simulink model "Vorlage_Anlagenteil_Pruefen_Jaehocha"  (R2021b)
settings: Solver=ode3  StartTime=0.0  StopTime=50  FixedStep=0.01  RelTol=1e-3
StopFcn:
  | clear con
model workspace (MAT data in the model file):
  A : Simulink.Signal (value not decoded)
undefined symbols (not defined in the file): sigbuilder_block
libraries: simulink x10, simulink_extras x7, aerolibanimutils x1
(part 2 of 2)

== system Vorlage_Anlagenteil_Pruefen_Jaehocha/Systemtest Simulation1/2_rot_mit_Deckel/Signal Builder10 ==
  Demux : Demux  Tag=STV Demux  Outputs=8
      settings: DisplayOption=none
  FromWs : FromWorkspace  Tag=STV FromWs  VariableName=tuvar
      SigBuilderData=|
      | common.afterFinalStr = 'Extrapolate'
      | common.sampleTime = 0
      | dataSet.timeRange = [0 11]
      | dataSet.name = 'Group 1'
      | sbobj.Groups.Name = 'Group 1'
      | sbobj.Groups.Signals(1).Name = 'aufzug_abwaerts'
      | sbobj.Groups.Signals(1).XData = [0 6 6 10.5 10.5 11]
      | sbobj.Groups.Signals(1).YData = [0 0 1 1 0 0]
      | sbobj.Groups.Signals(2).Name = 'aufzug_aufwaerts'
      | sbobj.Groups.Signals(2).XData = [0 0.5 0.5 5 5 11]
      | sbobj.Groups.Signals(2).YData = [0 0 1 1 0 0]
      | sbobj.Groups.Signals(3).Name = 'zylinder_ausschieben'
      | sbobj.Groups.Signals(3).XData = [0 5.5 5.5 6.2 6.2 11]
      | sbobj.Groups.Signals(3).YData = [0 0 1 1 0 0]
      | sbobj.Groups.Signals(4).Name = 'luft_an'
      | sbobj.Groups.Signals(4).XData = [0 5.5 5.5 7.5 7.5 11]
      | sbobj.Groups.Signals(4).YData = [0 0 1 1 0 0]
      | sbobj.Groups.Signals(5).Name = 'Signal 5'
      | sbobj.Groups.Signals(5).XData = [0 11]
      | sbobj.Groups.Signals(5).YData = [0 0]
      | sbobj.Groups.Signals(6).Name = 'Signal 6'
      | sbobj.Groups.Signals(6).XData = [0 11]
      | sbobj.Groups.Signals(6).YData = [0 0]
      | sbobj.Groups.Signals(7).Name = 'Signal 7'
      | sbobj.Groups.Signals(7).XData = [0 11]
      | sbobj.Groups.Signals(7).YData = [0 0]
      | sbobj.Groups.Signals(8).Name = 'station_frei'
      | sbobj.Groups.Signals(8).XData = [0 0.1 0.1 11]
      | sbobj.Groups.Signals(8).YData = [1 1 0 0]
      | sbobj.Groups.TimeRange = [0 11]
  aufzug_abwaerts : Outport  Tag=STV Outport  VectorParamsAs1DForOutWhenUnconnected=off
  aufzug_aufwaerts : Outport  Tag=STV Outport  Port=2  VectorParamsAs1DForOutWhenUnconnected=off
  zylinder_ausschieben : Outport  Tag=STV Outport  Port=3  VectorParamsAs1DForOutWhenUnconnected=off
  luft_an : Outport  Tag=STV Outport  Port=4  VectorParamsAs1DForOutWhenUnconnected=off
  Signal 5 : Outport  Tag=STV Outport  Port=5  VectorParamsAs1DForOutWhenUnconnected=off
  Signal 6 : Outport  Tag=STV Outport  Port=6  VectorParamsAs1DForOutWhenUnconnected=off
  Signal 7 : Outport  Tag=STV Outport  Port=7  VectorParamsAs1DForOutWhenUnconnected=off
  station_frei : Outport  Tag=STV Outport  Port=8  VectorParamsAs1DForOutWhenUnconnected=off
  wires:
  Demux/1 -> aufzug_abwaerts/1
  FromWs/1 -> Demux/1
  Demux/2 -> aufzug_aufwaerts/1
  Demux/3 -> zylinder_ausschieben/1
  Demux/4 -> luft_an/1
  Demux/5 -> Signal 5/1
  Demux/6 -> Signal 6/1
  Demux/7 -> Signal 7/1
  Demux/8 -> station_frei/1

== system Vorlage_Anlagenteil_Pruefen_Jaehocha/Systemtest Simulation1/2_rot_mit_Deckel/Signal Builder4 ==
  Demux : Demux  Tag=STV Demux  Outputs=6
      settings: DisplayOption=none
  FromWs : FromWorkspace  Tag=STV FromWs  VariableName=tuvar
      SigBuilderData=|
      | common.afterFinalStr = 'Extrapolate'
      | common.sampleTime = 0
      | dataSet.timeRange = [0 11]
      | dataSet.name = 'Group 1'
      | sbobj.Groups.Name = 'Group 1'
      | sbobj.Groups.Signals(1).Name = 'zylinder_platziert'
      | sbobj.Groups.Signals(1).XData = [0 0.3 0.3 11]
      | sbobj.Groups.Signals(1).YData = [1 1 0 0]
      | sbobj.Groups.Signals(2).Name = 'zylinder_schwarz'
      | sbobj.Groups.Signals(2).XData = [0 11]
      | sbobj.Groups.Signals(2).YData = [0 0]
      | sbobj.Groups.Signals(3).Name = 'zylinder_hoehe'
      | sbobj.Groups.Signals(3).XData = [0 5 5 5.6 5.6 11]
      | sbobj.Groups.Signals(3).YData = [0 0 28 28 0 0]
      | sbobj.Groups.Signals(4).Name = 'arbeitsraum_frei'
      | sbobj.Groups.Signals(4).XData = [0 0.5 0.5 10.5 10.5 10.8 10.8 11]
      | sbobj.Groups.Signals(4).YData = [1 1 0 0 1 1 0 0]
      | sbobj.Groups.Signals(5).Name = 'zylinder_entfernt_folge'
      | sbobj.Groups.Signals(5).XData = [0 10 10 10.5 10.5 11]
      | sbobj.Groups.Signals(5).YData = [0 0 1 1 0 0]
      | sbobj.Groups.Signals(6).Name = 'folge_belegt'
      | sbobj.Groups.Signals(6).XData = [0 4 5.5 11]
      | sbobj.Groups.Signals(6).YData = [0 0 0 0]
      | sbobj.Groups.TimeRange = [0 11]
  zylinder_platziert : Outport  Tag=STV Outport  VectorParamsAs1DForOutWhenUnconnected=off
  zylinder_schwarz : Outport  Tag=STV Outport  Port=2  VectorParamsAs1DForOutWhenUnconnected=off
  zylinder_hoehe : Outport  Tag=STV Outport  Port=3  VectorParamsAs1DForOutWhenUnconnected=off
  arbeitsraum_frei : Outport  Tag=STV Outport  Port=4  VectorParamsAs1DForOutWhenUnconnected=off
  zylinder_entfernt_folge : Outport  Tag=STV Outport  Port=5  VectorParamsAs1DForOutWhenUnconnected=off
  folge_belegt : Outport  Tag=STV Outport  Port=6  VectorParamsAs1DForOutWhenUnconnected=off
  wires:
  Demux/1 -> zylinder_platziert/1
  FromWs/1 -> Demux/1
  Demux/2 -> zylinder_schwarz/1
  Demux/3 -> zylinder_hoehe/1
  Demux/4 -> arbeitsraum_frei/1
  Demux/5 -> zylinder_entfernt_folge/1
  Demux/6 -> folge_belegt/1

== system Vorlage_Anlagenteil_Pruefen_Jaehocha/Systemtest Simulation1/2_rot_mit_Deckel/arbeitsraum_frei ==
  Add : Sum  Inputs=++++
  Constant : Constant
  Constant1 : Constant  Value=-1
  Constant2 : Constant
  Constant3 : Constant  Value=-1
  Data Type Conversion : DataTypeConversion  OutDataTypeStr=boolean
  Delay : Delay  DelayLength=0
  Delay1 : Delay  DelayLength=200
  Delay2 : Delay  DelayLength=1050
  Delay3 : Delay  DelayLength=1080
  Out1 : Outport  VectorParamsAs1DForOutWhenUnconnected=off
  wires:
  Constant/1 -> Delay/1
  Constant1/1 -> Delay1/1
  Delay/1 -> Add/1
  Delay1/1 -> Add/2
  Add/1 -> Data Type Conversion/1
  Data Type Conversion/1 -> Out1/1
  Constant2/1 -> Delay2/1
  Delay2/1 -> Add/3
  Constant3/1 -> Delay3/1
  Delay3/1 -> Add/4

== system Vorlage_Anlagenteil_Pruefen_Jaehocha/Systemtest Simulation1/2_rot_mit_Deckel/aufzug_abwaerts ==
  Add : Sum
  Constant : Constant
  Constant1 : Constant  Value=-1
  Data Type Conversion : DataTypeConversion  OutDataTypeStr=boolean
  Delay : Delay  DelayLength=600
  Delay1 : Delay  DelayLength=1050
  Out1 : Outport  VectorParamsAs1DForOutWhenUnconnected=off
  wires:
  Constant/1 -> Delay/1
  Constant1/1 -> Delay1/1
  Delay/1 -> Add/1
  Delay1/1 -> Add/2
  Add/1 -> Data Type Conversion/1
  Data Type Conversion/1 -> Out1/1

== system Vorlage_Anlagenteil_Pruefen_Jaehocha/Systemtest Simulation1/2_rot_mit_Deckel/aufzug_aufwaerts ==
  Add : Sum
  Constant : Constant
  Constant1 : Constant  Value=-1
  Data Type Conversion : DataTypeConversion  OutDataTypeStr=boolean
  Delay : Delay  DelayLength=50
  Delay1 : Delay  DelayLength=500
  Out1 : Outport  VectorParamsAs1DForOutWhenUnconnected=off
  wires:
  Constant/1 -> Delay/1
  Constant1/1 -> Delay1/1
  Delay/1 -> Add/1
  Delay1/1 -> Add/2
  Add/1 -> Data Type Conversion/1
  Data Type Conversion/1 -> Out1/1

== system Vorlage_Anlagenteil_Pruefen_Jaehocha/Systemtest Simulation1/2_rot_mit_Deckel/done_signal ==
  Constant : Constant
  Data Type Conversion : DataTypeConversion  OutDataTypeStr=boolean
  Delay : Delay  DelayLength=1080
  Out1 : Outport  VectorParamsAs1DForOutWhenUnconnected=off
  wires:
  Constant/1 -> Delay/1
  Data Type Conversion/1 -> Out1/1
  Delay/1 -> Data Type Conversion/1

== system Vorlage_Anlagenteil_Pruefen_Jaehocha/Systemtest Simulation1/2_rot_mit_Deckel/folge_belegt ==
  Constant : Constant  Value=0
  Data Type Conversion : DataTypeConversion  OutDataTypeStr=boolean
  Out1 : Outport  VectorParamsAs1DForOutWhenUnconnected=off
  wires:
  Constant/1 -> Data Type Conversion/1
  Data Type Conversion/1 -> Out1/1

== system Vorlage_Anlagenteil_Pruefen_Jaehocha/Systemtest Simulation1/2_rot_mit_Deckel/luft_an ==
  Add : Sum
  Constant : Constant
  Constant1 : Constant  Value=-1
  Data Type Conversion : DataTypeConversion  OutDataTypeStr=boolean
  Delay : Delay  DelayLength=550
  Delay1 : Delay  DelayLength=750
  Out1 : Outport  VectorParamsAs1DForOutWhenUnconnected=off
  wires:
  Constant/1 -> Delay/1
  Constant1/1 -> Delay1/1
  Delay/1 -> Add/1
  Delay1/1 -> Add/2
  Add/1 -> Data Type Conversion/1
  Data Type Conversion/1 -> Out1/1

== system Vorlage_Anlagenteil_Pruefen_Jaehocha/Systemtest Simulation1/2_rot_mit_Deckel/out5 ==
  Add : Sum
  Constant : Constant
  Constant1 : Constant  Value=-1
  Data Type Conversion : DataTypeConversion  OutDataTypeStr=boolean
  Delay : Delay  DelayLength=0
  Delay1 : Delay  DelayLength=0
  Out1 : Outport  VectorParamsAs1DForOutWhenUnconnected=off
  wires:
  Constant/1 -> Delay/1
  Constant1/1 -> Delay1/1
  Delay/1 -> Add/1
  Delay1/1 -> Add/2
  Add/1 -> Data Type Conversion/1
  Data Type Conversion/1 -> Out1/1

== system Vorlage_Anlagenteil_Pruefen_Jaehocha/Systemtest Simulation1/2_rot_mit_Deckel/out6 ==
  Add : Sum
  Constant : Constant
  Constant1 : Constant  Value=-1
  Data Type Conversion : DataTypeConversion  OutDataTypeStr=boolean
  Delay : Delay  DelayLength=0
  Delay1 : Delay  DelayLength=0
  Out1 : Outport  VectorParamsAs1DForOutWhenUnconnected=off
  wires:
  Constant/1 -> Delay/1
  Constant1/1 -> Delay1/1
  Delay/1 -> Add/1
  Delay1/1 -> Add/2
  Add/1 -> Data Type Conversion/1
  Data Type Conversion/1 -> Out1/1

== system Vorlage_Anlagenteil_Pruefen_Jaehocha/Systemtest Simulation1/2_rot_mit_Deckel/out7 ==
  Add : Sum
  Constant : Constant
  Constant1 : Constant  Value=-1
  Data Type Conversion : DataTypeConversion  OutDataTypeStr=boolean
  Delay : Delay  DelayLength=0
  Delay1 : Delay  DelayLength=0
  Out1 : Outport  VectorParamsAs1DForOutWhenUnconnected=off
  wires:
  Constant/1 -> Delay/1
  Constant1/1 -> Delay1/1
  Delay/1 -> Add/1
  Delay1/1 -> Add/2
  Add/1 -> Data Type Conversion/1
  Data Type Conversion/1 -> Out1/1

== system Vorlage_Anlagenteil_Pruefen_Jaehocha/Systemtest Simulation1/2_rot_mit_Deckel/station_frei ==
  Add : Sum
  Constant : Constant
  Constant1 : Constant  Value=-1
  Data Type Conversion : DataTypeConversion  OutDataTypeStr=boolean
  Delay : Delay  DelayLength=0
  Delay1 : Delay  DelayLength=10
  Out1 : Outport  VectorParamsAs1DForOutWhenUnconnected=off
  wires:
  Constant/1 -> Delay/1
  Constant1/1 -> Delay1/1
  Delay/1 -> Add/1
  Delay1/1 -> Add/2
  Add/1 -> Data Type Conversion/1
  Data Type Conversion/1 -> Out1/1

== system Vorlage_Anlagenteil_Pruefen_Jaehocha/Systemtest Simulation1/2_rot_mit_Deckel/zylinder_ausschieben ==
  Add : Sum
  Constant : Constant
  Constant1 : Constant  Value=-1
  Data Type Conversion : DataTypeConversion  OutDataTypeStr=boolean
  Delay : Delay  DelayLength=550
  Delay1 : Delay  DelayLength=620
  Out1 : Outport  VectorParamsAs1DForOutWhenUnconnected=off
  wires:
  Constant/1 -> Delay/1
  Constant1/1 -> Delay1/1
  Delay/1 -> Add/1
  Delay1/1 -> Add/2
  Add/1 -> Data Type Conversion/1
  Data Type Conversion/1 -> Out1/1

== system Vorlage_Anlagenteil_Pruefen_Jaehocha/Systemtest Simulation1/2_rot_mit_Deckel/zylinder_entfernt_folge ==
  Add : Sum
  Constant : Constant
  Constant1 : Constant  Value=-1
  Data Type Conversion : DataTypeConversion  OutDataTypeStr=boolean
  Delay : Delay  DelayLength=1000
  Delay1 : Delay  DelayLength=1050
  Out1 : Outport  VectorParamsAs1DForOutWhenUnconnected=off
  wires:
  Constant/1 -> Delay/1
  Constant1/1 -> Delay1/1
  Delay/1 -> Add/1
  Delay1/1 -> Add/2
  Add/1 -> Data Type Conversion/1
  Data Type Conversion/1 -> Out1/1

== system Vorlage_Anlagenteil_Pruefen_Jaehocha/Systemtest Simulation1/2_rot_mit_Deckel/zylinder_hoehe ==
  Add : Sum
  Constant : Constant  Value=28
  Constant1 : Constant  Value=-28
  Delay : Delay  DelayLength=50
  Delay1 : Delay  DelayLength=900
  Out1 : Outport  VectorParamsAs1DForOutWhenUnconnected=off
  wires:
  Constant/1 -> Delay/1
  Constant1/1 -> Delay1/1
  Delay/1 -> Add/1
  Delay1/1 -> Add/2
  Add/1 -> Out1/1

== system Vorlage_Anlagenteil_Pruefen_Jaehocha/Systemtest Simulation1/2_rot_mit_Deckel/zylinder_platziert ==
  Add : Sum
  Constant : Constant
  Constant1 : Constant  Value=-1
  Data Type Conversion : DataTypeConversion  OutDataTypeStr=boolean
  Delay : Delay  DelayLength=0
  Delay1 : Delay  DelayLength=30
  Out1 : Outport  VectorParamsAs1DForOutWhenUnconnected=off
  wires:
  Constant/1 -> Delay/1
  Constant1/1 -> Delay1/1
  Delay/1 -> Add/1
  Delay1/1 -> Add/2
  Add/1 -> Data Type Conversion/1
  Data Type Conversion/1 -> Out1/1

== system Vorlage_Anlagenteil_Pruefen_Jaehocha/Systemtest Simulation1/2_rot_mit_Deckel/zylinder_schwarz ==
  Add : Sum
  Constant : Constant
  Constant1 : Constant  Value=-1
  Data Type Conversion : DataTypeConversion  OutDataTypeStr=boolean
  Delay : Delay  DelayLength=0
  Delay1 : Delay  DelayLength=0
  Out1 : Outport  VectorParamsAs1DForOutWhenUnconnected=off
  wires:
  Constant/1 -> Delay/1
  Constant1/1 -> Delay1/1
  Delay/1 -> Add/1
  Delay1/1 -> Add/2
  Add/1 -> Data Type Conversion/1
  Data Type Conversion/1 -> Out1/1

== system Vorlage_Anlagenteil_Pruefen_Jaehocha/Systemtest Simulation1/3_rot_ohne_Deckel/Signal Builder10 ==
  Demux : Demux  Tag=STV Demux  Outputs=8
      settings: DisplayOption=none
  FromWs : FromWorkspace  Tag=STV FromWs  VariableName=tuvar
      SigBuilderData=|
      | common.afterFinalStr = 'Extrapolate'
      | common.sampleTime = 0
      | dataSet.timeRange = [0 11]
      | dataSet.name = 'Group 1'
      | sbobj.Groups.Name = 'Group 1'
      | sbobj.Groups.Signals(1).Name = 'aufzug_abwaerts'
      | sbobj.Groups.Signals(1).XData = [0 5.5 5.5 10 10 11]
      | sbobj.Groups.Signals(1).YData = [0 0 1 1 0 0]
      | sbobj.Groups.Signals(2).Name = 'aufzug_aufwaerts'
      | sbobj.Groups.Signals(2).XData = [0 0.5 0.5 5 5 11]
      | sbobj.Groups.Signals(2).YData = [0 0 1 1 0 0]
      | sbobj.Groups.Signals(3).Name = 'zylinder_ausschieben'
      | sbobj.Groups.Signals(3).XData = [0 10 10 10.48 10.48 11]
      | sbobj.Groups.Signals(3).YData = [0 0 1 1 0 0]
      | sbobj.Groups.Signals(4).Name = 'luft_an'
      | sbobj.Groups.Signals(4).XData = [0 7.5 11]
      | sbobj.Groups.Signals(4).YData = [0 0 0]
      | sbobj.Groups.Signals(5).Name = 'Signal 5'
      | sbobj.Groups.Signals(5).XData = [0 11]
      | sbobj.Groups.Signals(5).YData = [0 0]
      | sbobj.Groups.Signals(6).Name = 'Signal 6'
      | sbobj.Groups.Signals(6).XData = [0 11]
      | sbobj.Groups.Signals(6).YData = [0 0]
      | sbobj.Groups.Signals(7).Name = 'Signal 7'
      | sbobj.Groups.Signals(7).XData = [0 11]
      | sbobj.Groups.Signals(7).YData = [0 0]
      | sbobj.Groups.Signals(8).Name = 'station_frei'
      | sbobj.Groups.Signals(8).XData = [0 0.1 0.1 11]
      | sbobj.Groups.Signals(8).YData = [1 1 0 0]
      | sbobj.Groups.TimeRange = [0 11]
  aufzug_abwaerts : Outport  Tag=STV Outport  VectorParamsAs1DForOutWhenUnconnected=off
  aufzug_aufwaerts : Outport  Tag=STV Outport  Port=2  VectorParamsAs1DForOutWhenUnconnected=off
  zylinder_ausschieben : Outport  Tag=STV Outport  Port=3  VectorParamsAs1DForOutWhenUnconnected=off
  luft_an : Outport  Tag=STV Outport  Port=4  VectorParamsAs1DForOutWhenUnconnected=off
  Signal 5 : Outport  Tag=STV Outport  Port=5  VectorParamsAs1DForOutWhenUnconnected=off
  Signal 6 : Outport  Tag=STV Outport  Port=6  VectorParamsAs1DForOutWhenUnconnected=off
  Signal 7 : Outport  Tag=STV Outport  Port=7  VectorParamsAs1DForOutWhenUnconnected=off
  station_frei : Outport  Tag=STV Outport  Port=8  VectorParamsAs1DForOutWhenUnconnected=off
  wires:
  Demux/1 -> aufzug_abwaerts/1
  FromWs/1 -> Demux/1
  Demux/2 -> aufzug_aufwaerts/1
  Demux/3 -> zylinder_ausschieben/1
  Demux/4 -> luft_an/1
  Demux/5 -> Signal 5/1
  Demux/6 -> Signal 6/1
  Demux/7 -> Signal 7/1
  Demux/8 -> station_frei/1

== system Vorlage_Anlagenteil_Pruefen_Jaehocha/Systemtest Simulation1/3_rot_ohne_Deckel/Signal Builder4 ==
  Demux : Demux  Tag=STV Demux  Outputs=6
      settings: DisplayOption=none
  FromWs : FromWorkspace  Tag=STV FromWs  VariableName=tuvar
      SigBuilderData=|
      | common.afterFinalStr = 'Extrapolate'
      | common.sampleTime = 0
      | dataSet.timeRange = [0 11]
      | dataSet.name = 'Group 1'
      | sbobj.Groups.Name = 'Group 1'
      | sbobj.Groups.Signals(1).Name = 'zylinder_platziert'
      | sbobj.Groups.Signals(1).XData = [0 0.3 0.3 11]
      | sbobj.Groups.Signals(1).YData = [1 1 0 0]
      | sbobj.Groups.Signals(2).Name = 'zylinder_schwarz'
      | sbobj.Groups.Signals(2).XData = [0 11]
      | sbobj.Groups.Signals(2).YData = [0 0]
      | sbobj.Groups.Signals(3).Name = 'zylinder_hoehe'
      | sbobj.Groups.Signals(3).XData = [0 5 5 5.6 5.6 11]
      | sbobj.Groups.Signals(3).YData = [0 0 25 25 0 0]
      | sbobj.Groups.Signals(4).Name = 'arbeitsraum_frei'
      | sbobj.Groups.Signals(4).XData = [0 0.5 0.5 10 10 10.8 10.8 11]
      | sbobj.Groups.Signals(4).YData = [1 1 0 0 1 1 0 0]
      | sbobj.Groups.Signals(5).Name = 'zylinder_entfernt_folge'
      | sbobj.Groups.Signals(5).XData = [0 10 10.5 11]
      | sbobj.Groups.Signals(5).YData = [0 0 0 0]
      | sbobj.Groups.Signals(6).Name = 'folge_belegt'
      | sbobj.Groups.Signals(6).XData = [0 4 5.5 11]
      | sbobj.Groups.Signals(6).YData = [0 0 0 0]
      | sbobj.Groups.TimeRange = [0 11]
  zylinder_platziert : Outport  Tag=STV Outport  VectorParamsAs1DForOutWhenUnconnected=off
  zylinder_schwarz : Outport  Tag=STV Outport  Port=2  VectorParamsAs1DForOutWhenUnconnected=off
  zylinder_hoehe : Outport  Tag=STV Outport  Port=3  VectorParamsAs1DForOutWhenUnconnected=off
  arbeitsraum_frei : Outport  Tag=STV Outport  Port=4  VectorParamsAs1DForOutWhenUnconnected=off
  zylinder_entfernt_folge : Outport  Tag=STV Outport  Port=5  VectorParamsAs1DForOutWhenUnconnected=off
  folge_belegt : Outport  Tag=STV Outport  Port=6  VectorParamsAs1DForOutWhenUnconnected=off
  wires:
  Demux/1 -> zylinder_platziert/1
  FromWs/1 -> Demux/1
  Demux/2 -> zylinder_schwarz/1
  Demux/3 -> zylinder_hoehe/1
  Demux/4 -> arbeitsraum_frei/1
  Demux/5 -> zylinder_entfernt_folge/1
  Demux/6 -> folge_belegt/1

== system Vorlage_Anlagenteil_Pruefen_Jaehocha/Systemtest Simulation1/3_rot_ohne_Deckel/arbeitsraum_frei ==
  Add : Sum  Inputs=++++
  Constant : Constant
  Constant1 : Constant  Value=-1
  Constant2 : Constant
  Constant3 : Constant  Value=-1
  Data Type Conversion : DataTypeConversion  OutDataTypeStr=boolean
  Delay : Delay  DelayLength=0
  Delay1 : Delay  DelayLength=200
  Delay2 : Delay  DelayLength=1000
  Delay3 : Delay  DelayLength=1080
  Out1 : Outport  VectorParamsAs1DForOutWhenUnconnected=off
  wires:
  Constant/1 -> Delay/1
  Constant1/1 -> Delay1/1
  Delay/1 -> Add/1
  Delay1/1 -> Add/2
  Add/1 -> Data Type Conversion/1
  Data Type Conversion/1 -> Out1/1
  Constant2/1 -> Delay2/1
  Delay2/1 -> Add/3
  Constant3/1 -> Delay3/1
  Delay3/1 -> Add/4

== system Vorlage_Anlagenteil_Pruefen_Jaehocha/Systemtest Simulation1/3_rot_ohne_Deckel/aufzug_abwaerts ==
  Add : Sum
  Constant : Constant
  Constant1 : Constant  Value=-1
  Data Type Conversion : DataTypeConversion  OutDataTypeStr=boolean
  Delay : Delay  DelayLength=550
  Delay1 : Delay  DelayLength=1000
  Out1 : Outport  VectorParamsAs1DForOutWhenUnconnected=off
  wires:
  Constant/1 -> Delay/1
  Constant1/1 -> Delay1/1
  Delay/1 -> Add/1
  Delay1/1 -> Add/2
  Add/1 -> Data Type Conversion/1
  Data Type Conversion/1 -> Out1/1

== system Vorlage_Anlagenteil_Pruefen_Jaehocha/Systemtest Simulation1/3_rot_ohne_Deckel/aufzug_aufwaerts ==
  Add : Sum
  Constant : Constant
  Constant1 : Constant  Value=-1
  Data Type Conversion : DataTypeConversion  OutDataTypeStr=boolean
  Delay : Delay  DelayLength=50
  Delay1 : Delay  DelayLength=500
  Out1 : Outport  VectorParamsAs1DForOutWhenUnconnected=off
  wires:
  Constant/1 -> Delay/1
  Constant1/1 -> Delay1/1
  Delay/1 -> Add/1
  Delay1/1 -> Add/2
  Add/1 -> Data Type Conversion/1
  Data Type Conversion/1 -> Out1/1

== system Vorlage_Anlagenteil_Pruefen_Jaehocha/Systemtest Simulation1/3_rot_ohne_Deckel/folge_belegt ==
  Constant : Constant  Value=0
  Data Type Conversion : DataTypeConversion  OutDataTypeStr=boolean
  Out1 : Outport  VectorParamsAs1DForOutWhenUnconnected=off
  wires:
  Constant/1 -> Data Type Conversion/1
  Data Type Conversion/1 -> Out1/1

== system Vorlage_Anlagenteil_Pruefen_Jaehocha/Systemtest Simulation1/3_rot_ohne_Deckel/luft_an ==
  Add : Sum
  Constant : Constant
  Constant1 : Constant  Value=-1
  Data Type Conversion : DataTypeConversion  OutDataTypeStr=boolean
  Delay : Delay  DelayLength=0
  Delay1 : Delay  DelayLength=0
  Out1 : Outport  VectorParamsAs1DForOutWhenUnconnected=off
  wires:
  Constant/1 -> Delay/1
  Constant1/1 -> Delay1/1
  Delay/1 -> Add/1
  Delay1/1 -> Add/2
  Add/1 -> Data Type Conversion/1
  Data Type Conversion/1 -> Out1/1

== system Vorlage_Anlagenteil_Pruefen_Jaehocha/Systemtest Simulation1/3_rot_ohne_Deckel/out5 ==
  Add : Sum
  Constant : Constant
  Constant1 : Constant  Value=-1
  Data Type Conversion : DataTypeConversion  OutDataTypeStr=boolean
  Delay : Delay  DelayLength=0
  Delay1 : Delay  DelayLength=0
  Out1 : Outport  VectorParamsAs1DForOutWhenUnconnected=off
  wires:
  Constant/1 -> Delay/1
  Constant1/1 -> Delay1/1
  Delay/1 -> Add/1
  Delay1/1 -> Add/2
  Add/1 -> Data Type Conversion/1
  Data Type Conversion/1 -> Out1/1

== system Vorlage_Anlagenteil_Pruefen_Jaehocha/Systemtest Simulation1/3_rot_ohne_Deckel/out6 ==
  Add : Sum
  Constant : Constant
  Constant1 : Constant  Value=-1
  Data Type Conversion : DataTypeConversion  OutDataTypeStr=boolean
  Delay : Delay  DelayLength=0
  Delay1 : Delay  DelayLength=0
  Out1 : Outport  VectorParamsAs1DForOutWhenUnconnected=off
  wires:
  Constant/1 -> Delay/1
  Constant1/1 -> Delay1/1
  Delay/1 -> Add/1
  Delay1/1 -> Add/2
  Add/1 -> Data Type Conversion/1
  Data Type Conversion/1 -> Out1/1

== system Vorlage_Anlagenteil_Pruefen_Jaehocha/Systemtest Simulation1/3_rot_ohne_Deckel/out7 ==
  Add : Sum
  Constant : Constant
  Constant1 : Constant  Value=-1
  Data Type Conversion : DataTypeConversion  OutDataTypeStr=boolean
  Delay : Delay  DelayLength=0
  Delay1 : Delay  DelayLength=0
  Out1 : Outport  VectorParamsAs1DForOutWhenUnconnected=off
  wires:
  Constant/1 -> Delay/1
  Constant1/1 -> Delay1/1
  Delay/1 -> Add/1
  Delay1/1 -> Add/2
  Add/1 -> Data Type Conversion/1
  Data Type Conversion/1 -> Out1/1

== system Vorlage_Anlagenteil_Pruefen_Jaehocha/Systemtest Simulation1/3_rot_ohne_Deckel/station_frei ==
  Add : Sum
  Constant : Constant
  Constant1 : Constant  Value=-1
  Data Type Conversion : DataTypeConversion  OutDataTypeStr=boolean
  Delay : Delay  DelayLength=0
  Delay1 : Delay  DelayLength=10
  Out1 : Outport  VectorParamsAs1DForOutWhenUnconnected=off
  wires:
  Constant/1 -> Delay/1
  Constant1/1 -> Delay1/1
  Delay/1 -> Add/1
  Delay1/1 -> Add/2
  Add/1 -> Data Type Conversion/1
  Data Type Conversion/1 -> Out1/1

== system Vorlage_Anlagenteil_Pruefen_Jaehocha/Systemtest Simulation1/3_rot_ohne_Deckel/zylinder_ausschieben ==
  Add : Sum
  Constant : Constant
  Constant1 : Constant  Value=-1
  Data Type Conversion : DataTypeConversion  OutDataTypeStr=boolean
  Delay : Delay  DelayLength=1000
  Delay1 : Delay  DelayLength=1050
  Out1 : Outport  VectorParamsAs1DForOutWhenUnconnected=off
  wires:
  Constant/1 -> Delay/1
  Constant1/1 -> Delay1/1
  Delay/1 -> Add/1
  Delay1/1 -> Add/2
  Add/1 -> Data Type Conversion/1
  Data Type Conversion/1 -> Out1/1

== system Vorlage_Anlagenteil_Pruefen_Jaehocha/Systemtest Simulation1/3_rot_ohne_Deckel/zylinder_entfernt_folge ==
  Add : Sum
  Constant : Constant
  Constant1 : Constant  Value=-1
  Data Type Conversion : DataTypeConversion  OutDataTypeStr=boolean
  Delay : Delay  DelayLength=0
  Delay1 : Delay  DelayLength=0
  Out1 : Outport  VectorParamsAs1DForOutWhenUnconnected=off
  wires:
  Constant/1 -> Delay/1
  Constant1/1 -> Delay1/1
  Delay/1 -> Add/1
  Delay1/1 -> Add/2
  Add/1 -> Data Type Conversion/1
  Data Type Conversion/1 -> Out1/1

== system Vorlage_Anlagenteil_Pruefen_Jaehocha/Systemtest Simulation1/3_rot_ohne_Deckel/zylinder_hoehe ==
  Add : Sum
  Constant : Constant  Value=25
  Constant1 : Constant  Value=-25
  Delay : Delay  DelayLength=50
  Delay1 : Delay  DelayLength=900
  Out1 : Outport  VectorParamsAs1DForOutWhenUnconnected=off
  wires:
  Constant/1 -> Delay/1
  Constant1/1 -> Delay1/1
  Delay/1 -> Add/1
  Delay1/1 -> Add/2
  Add/1 -> Out1/1

== system Vorlage_Anlagenteil_Pruefen_Jaehocha/Systemtest Simulation1/3_rot_ohne_Deckel/zylinder_platziert ==
  Add : Sum
  Constant : Constant
  Constant1 : Constant  Value=-1
  Data Type Conversion : DataTypeConversion  OutDataTypeStr=boolean
  Delay : Delay  DelayLength=0
  Delay1 : Delay  DelayLength=30
  Out1 : Outport  VectorParamsAs1DForOutWhenUnconnected=off
  wires:
  Constant/1 -> Delay/1
  Constant1/1 -> Delay1/1
  Delay/1 -> Add/1
  Delay1/1 -> Add/2
  Add/1 -> Data Type Conversion/1
  Data Type Conversion/1 -> Out1/1

== system Vorlage_Anlagenteil_Pruefen_Jaehocha/Systemtest Simulation1/3_rot_ohne_Deckel/zylinder_schwarz ==
  Add : Sum
  Constant : Constant
  Constant1 : Constant  Value=-1
  Data Type Conversion : DataTypeConversion  OutDataTypeStr=boolean
  Delay : Delay  DelayLength=0
  Delay1 : Delay  DelayLength=0
  Out1 : Outport  VectorParamsAs1DForOutWhenUnconnected=off
  wires:
  Constant/1 -> Delay/1
  Constant1/1 -> Delay1/1
  Delay/1 -> Add/1
  Delay1/1 -> Add/2
  Add/1 -> Data Type Conversion/1
  Data Type Conversion/1 -> Out1/1

== stateflow chart Vorlage_Anlagenteil_Pruefen_Jaehocha/Steuerung ==
  state Anfang
    aufzug_abwaerts = 0;
    aufzug_aufwaerts =0;
    zylinder_ausschieben = 0;
    luft_an = 0;
    station_frei = 0;
    schritt = 0;
    %anfangszustand alle aktoren
    %sind ausgeschaltet
  state Pruefungszustand_anfang
    aufzug_aufwaerts = 1;
    schritt=3;
    %wenn Arbeitraum frei ist
    %Aufzug geht hoch
  state Freigabesignal_gegeben
    station_frei = 1;
    schritt = 1;
    %freigabesiganl gegeben
  state Werkstueck_erkennen
    station_frei = 0;
    schritt = 2;
    %werkstueck wird erkannt dann
    %station_frei wird wieder 0
  state Pruefungszustand_hoehen_und_farbe
    aufzug_aufwaerts = 0;
    schritt=4;
    %wenn Aufzug hoch gekommen,
    %Aktor von Aufzug_aufwaerts ausschaltet
    %bekommen Daten von Sensoren
  state Hebebuehne_position_initialisierung
    aufzug_abwaerts = 1;
    schritt=7;
    %aufzug geht unter
  state Pruefungszustand_mti_Deckel1
    zylinder_ausschieben = 0;
    luft_an = 0;
    schritt=6;
    %luft aus
    %Auschiebenzlinder wird eingezogen
  state Pruefungszustand_mti_Deckel
    zylinder_ausschieben = 1;
    luft_an = 1;
    schritt=5;
    %pruefszustand fuer zylinder mit Deckel
    %luft an
    %ausschiebenzylinder schiebt zylinder
  state Pruefungszustand_ohne_Deckel
    aufzug_abwaerts = 1;
    schritt=8;
    %pruefszustand fuer zylinder ohne deckel
    %Aufzug geht unter
  state Pruefungszustand_ohne_Deckel2
    zylinder_ausschieben = 0;
    schritt=10;
    %Ausschiebenzlinder wird eingezogen
  state Pruefungszustand_ohne_Deckel1
    zylinder_ausschieben = 1;
    aufzug_abwaerts = 0;
    schritt=9;
    %ausschiebenzylinder schiebt zylinder
    %aufzugsaktor wird aus
  (default) -> Anfang
  Pruefungszustand_ohne_Deckel2 -> Anfang : [zylinder_eingefahren == 1]
  Anfang -> Freigabesignal_gegeben : [(werkstueck_vorhanden == 0) & zylinder_eingefahren == 1 & aufzug_unten == 1]
  Werkstueck_erkennen -> Pruefungszustand_anfang : [arbeitsraum_frei == 1]{after(0.5,sec)}
  Freigabesignal_gegeben -> Werkstueck_erkennen : [werkstueck_vorhanden == 1]
  Hebebuehne_position_initialisierung -> Anfang : [aufzug_unten == 1]
  Pruefungszustand_anfang -> Pruefungszustand_hoehen_und_farbe : [aufzug_oben == 1]{after(1,sec)}
  Pruefungszustand_hoehen_und_farbe -> Pruefungszustand_mti_Deckel [order 1] : [((hoehe_ok ~= werkstueck_nicht_schwarz) == 1) && (folgestation_belegt == 0)]
  Pruefungszustand_mti_Deckel -> Pruefungszustand_mti_Deckel1 : after(2,sec)
  Pruefungszustand_mti_Deckel1 -> Hebebuehne_position_initialisierung : [zylinder_eingefahren == 1]
  Pruefungszustand_hoehen_und_farbe -> Pruefungszustand_ohne_Deckel [order 2] : [(hoehe_ok ~= werkstueck_nicht_schwarz) == 0]{after(1,sec)}
  Pruefungszustand_ohne_Deckel -> Pruefungszustand_ohne_Deckel1 : [aufzug_unten == 1]
  Pruefungszustand_ohne_Deckel1 -> Pruefungszustand_ohne_Deckel2 : after(2,sec)
  data: werkstueck_vorhanden input; werkstueck_nicht_schwarz input; arbeitsraum_frei input; hoehe_ok input; aufzug_oben input; aufzug_unten input; zylinder_eingefahren input; folgestation_belegt input; aufzug_abwaerts output; aufzug_aufwaerts output; zylinder_ausschieben output; luft_an output; station_frei output; schritt output

== matlab function Vorlage_Anlagenteil_Pruefen_Jaehocha/Write/Write1 ==
  data: step input; actuators input
function fcn (step, actuators)
coder.extrinsic('num2str')
coder.extrinsic('tcpclient')
coder.extrinsic('unicode2native')
coder.extrinsic('write')
coder.extrinsic('existsvar')
coder.extrinsic('evalin')
coder.extrinsic('assignin')

if(existsvar('base', 'con'))
    con = evalin('base', 'con');
else
    con = tcpclient('127.0.0.1', 4600);
    assignin('base', 'con', con);
end
word = controlword(actuators, step);
write(con, [unicode2native(num2str(word)), 10]);

== matlab function Vorlage_Anlagenteil_Pruefen_Jaehocha/Read/Read ==
  data: senarr output
function senarr = fcn()
coder.extrinsic('tcpclient')
coder.extrinsic('chararr2num')
coder.extrinsic('evalin')
coder.extrinsic('assignin')
coder.extrinsic('existsvar')
coder.extrinsic('read')

if(existsvar('base', 'con'))
    con = evalin('base', 'con');
else
    con = tcpclient('127.0.0.1', 4600); 
    assignin('base', 'con', con);
end
charlen = 20;
sensors = 0;
r = read(con, charlen);
sensors = chararr2num(r);
senarr = splitsignals(sensors);
